simulink model "Boomerang_Simulink_validation_smAoA"  (R2023a)
settings: Solver=ode4  StartTime=0.0  StopTime=t  FixedStep=dt  MaxStep=maxstep  MinStep=minstep
values from neighbouring files (symbols this model uses):
  c = 5e-2    (= 0.05)    [Boomerang_4Wings.m]    (also in Boomerang_4Wings_Titan.m = 0.0488; Boomerang_4Wings_Venus52.m; Boomerang_4Wings_Venus60.m = 0.065; Boomerang_Cropped_Validation.m = 0.0381)
  CDdata = [x_CD, y_CD]    [Boomerang_4Wings.m]    (also in Boomerang_4Wings_Titan.m; Boomerang_4Wings_Venus52.m; Boomerang_4Wings_Venus60.m; Boomerang_Cropped_Validation.m)
  CLdata = [x_CL, y_CL]    [Boomerang_4Wings.m]    (also in Boomerang_4Wings_Titan.m; Boomerang_4Wings_Venus52.m; Boomerang_4Wings_Venus60.m; Boomerang_Cropped_Validation.m)
  CMdata = [x_CM, y_CM]    [Boomerang_4Wings.m]    (also in Boomerang_4Wings_Titan.m; Boomerang_4Wings_Venus52.m; Boomerang_4Wings_Venus60.m; Boomerang_Cropped_Validation.m)
  Eul0 = [0; 0; 0]    [Boomerang_4Wings.m]    (also in Boomerang_4Wings_Titan.m; Boomerang_4Wings_Venus52.m; Boomerang_4Wings_Venus60.m; Boomerang_Cropped_Validation.m)
  g = 9.81    [Boomerang_4Wings.m]    (also in Boomerang_4Wings_Titan.m = 1.35; Boomerang_4Wings_Venus52.m; Boomerang_4Wings_Venus60.m = 8.87; Boomerang_Cropped_Validation.m)
  invJ = inv(J)    [Boomerang_4Wings.m]    (also in Boomerang_4Wings_Titan.m; Boomerang_4Wings_Venus52.m; Boomerang_4Wings_Venus60.m; Boomerang_Cropped_Validation.m)
  invm = inv(m)    [Boomerang_4Wings.m]    (also in Boomerang_4Wings_Titan.m; Boomerang_4Wings_Venus52.m; Boomerang_4Wings_Venus60.m; Boomerang_Cropped_Validation.m)
  invTI0 = transpose(TI0)    [AttitudePlot.m]    (also in AttitudePlot_V0.m = transpose(T); Boomerang_4Wings.m; Boomerang_4Wings_Titan.m; Boomerang_4Wings_Venus52.m)
  invTj = zeros(3,3,nw)    [Boomerang_4Wings.m]    (also in Boomerang_4Wings_Titan.m; Boomerang_4Wings_Venus52.m; Boomerang_4Wings_Venus60.m; Boomerang_Cropped_Validation.m)
  J = J + (Ji(:,:,i))    [Boomerang_4Wings.m]    (also in Boomerang_4Wings_Titan.m = diag(diag(J)); Boomerang_4Wings_Venus52.m; Boomerang_4Wings_Venus60.m; Boomerang_Cropped_Validation.m = [Ixx Ixy Ixz)
  l_integrate = linspace(0,l_blade,n)    [Boomerang_4Wings.m]    (also in Boomerang_4Wings_Titan.m; Boomerang_4Wings_Venus52.m; Boomerang_4Wings_Venus60.m; Boomerang_Cropped_Validation.m = linspace(l_blade_0,l_blade,n))
  m = m_b*eye(3) + m_add    [Boomerang_4Wings.m]    (also in Boomerang_4Wings_Titan.m; Boomerang_4Wings_Venus52.m; Boomerang_4Wings_Venus60.m; Boomerang_Cropped_Validation.m)
  nw = 4    [Boomerang_4Wings.m]    (also in Boomerang_4Wings_Titan.m; Boomerang_4Wings_Venus52.m; Boomerang_4Wings_Venus60.m; Boomerang_Cropped_Validation.m = 3)
  omega0 = [0; 0; 10*pi*2]    [Boomerang_4Wings.m]    (also in Boomerang_4Wings_Titan.m = [0; 0; r*pi*2]; Boomerang_4Wings_Venus52.m; Boomerang_4Wings_Venus60.m; Boomerang_Cropped_Validation.m = [0; 0; r])
  PHI0 = deg2rad(PHI0)    [AttitudePlot.m]    (also in AttitudePlot_V0.m; Boomerang_4Wings.m; Boomerang_4Wings_Titan.m; Boomerang_4Wings_Venus52.m)
  PSI0 = deg2rad(PSI0)    [AttitudePlot.m]    (also in AttitudePlot_V0.m; Boomerang_4Wings.m; Boomerang_4Wings_Titan.m; Boomerang_4Wings_Venus52.m)
  R_pos0 = [0; 0; 1.5]    [Boomerang_4Wings.m]    (also in Boomerang_4Wings_Titan.m; Boomerang_4Wings_Venus52.m; Boomerang_4Wings_Venus60.m; Boomerang_Cropped_Validation.m = [0; 0; 1.8])
  rho = 1.22    [Boomerang_4Wings.m]    (also in Boomerang_4Wings_Titan.m = 5.368; Boomerang_4Wings_Venus52.m = 1.3288004; Boomerang_4Wings_Venus60.m = 0.49007955; Boomerang_Cropped_Validation.m)
  S = pi*R^2    (= 0.196349540849)    [Boomerang_4Wings.m]    (also in Boomerang_4Wings_Titan.m = 0.228; Boomerang_4Wings_Venus52.m; Boomerang_4Wings_Venus60.m = 0.282743338823; Boomerang_Cropped_Validation.m = 0.0651440652648)
  THETA0 = deg2rad(THETA0)    [AttitudePlot.m]    (also in AttitudePlot_V0.m; Boomerang_4Wings.m; Boomerang_4Wings_Titan.m; Boomerang_4Wings_Venus52.m)
  thetaj = 0    [Boomerang_4Wings.m]    (also in Boomerang_4Wings_Titan.m; Boomerang_4Wings_Venus52.m; Boomerang_4Wings_Venus60.m; Boomerang_Cropped_Validation.m = deg2rad(thetaj))
  TI0 = RI01*RI02*RI03    [AttitudePlot.m]    (also in Boomerang_4Wings.m; Boomerang_4Wings_Titan.m; Boomerang_4Wings_Venus52.m; Boomerang_4Wings_Venus60.m)
  Tj = zeros(3,3, nw)    [Boomerang_4Wings.m]    (also in Boomerang_4Wings_Titan.m; Boomerang_4Wings_Venus52.m; Boomerang_4Wings_Venus60.m; Boomerang_Cropped_Validation.m)
  u0 = TI0*U0    [Boomerang_4Wings.m]    (also in Boomerang_4Wings_Titan.m; Boomerang_4Wings_Venus52.m; Boomerang_4Wings_Venus60.m; Boomerang_Cropped_Validation.m)
  v_wind = [0; 0; 0]    [Boomerang_4Wings.m]    (also in Boomerang_4Wings_Titan.m; Boomerang_4Wings_Venus52.m; Boomerang_4Wings_Venus60.m; Boomerang_Cropped_Validation.m)
  x_ac = zeros(3,nw)    [Boomerang_4Wings.m]    (also in Boomerang_4Wings_Titan.m = 0; Boomerang_4Wings_Venus52.m; Boomerang_4Wings_Venus60.m; Boomerang_Cropped_Validation.m)
libraries: simulink_extras x1
settings Model: Creator=dsantis  LastModifiedBy=dsantis

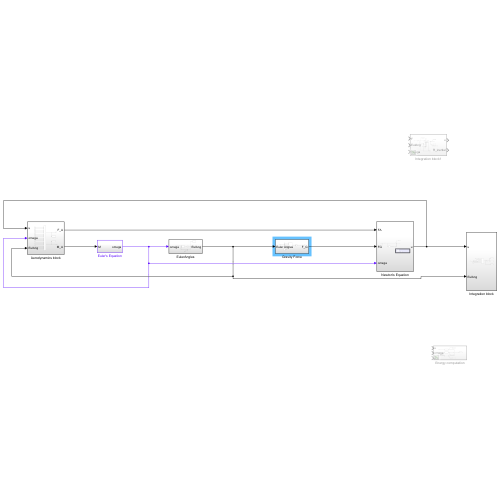
[thumbnail: Simulink's stored preview of the top-level diagram]
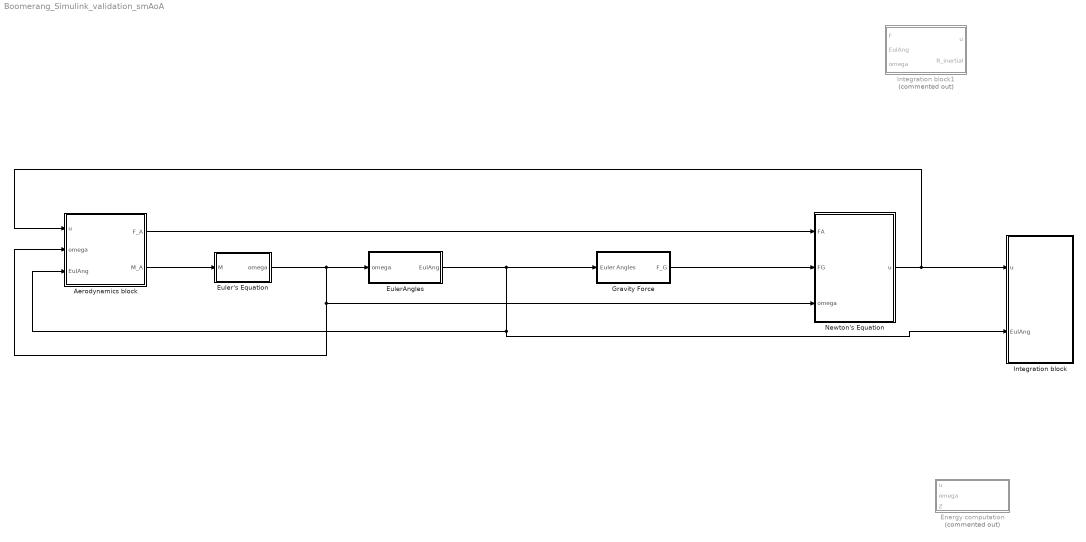
== system Boomerang_Simulink_validation_smAoA ==
  Aerodynamics block : Subsystem
  Energy computation : Subsystem  Commented=on
  Euler's Equation : Subsystem
  EulerAngles : Subsystem
  Gravity Force : Subsystem
  Integration block : Subsystem
  Integration block1 : Subsystem  Commented=on
  Newton's Equation : Subsystem
  wires:
  Euler's Equation/1(omega) -> EulerAngles/1(omega), Aerodynamics block/2(omega), Newton's Equation/3(omega)
  Newton's Equation/1(u) -> Aerodynamics block/1(u), Integration block/1(u)
  Gravity Force/1(F_G) -> Newton's Equation/2(FG)
  Aerodynamics block/2(M_A) -> Euler's Equation/1(M)
  EulerAngles/1(EulAng) -> Aerodynamics block/3(EulAng), Integration block/2(EulAng), Gravity Force/1(Euler Angles)
  Aerodynamics block/1(F_A) -> Newton's Equation/1(FA)

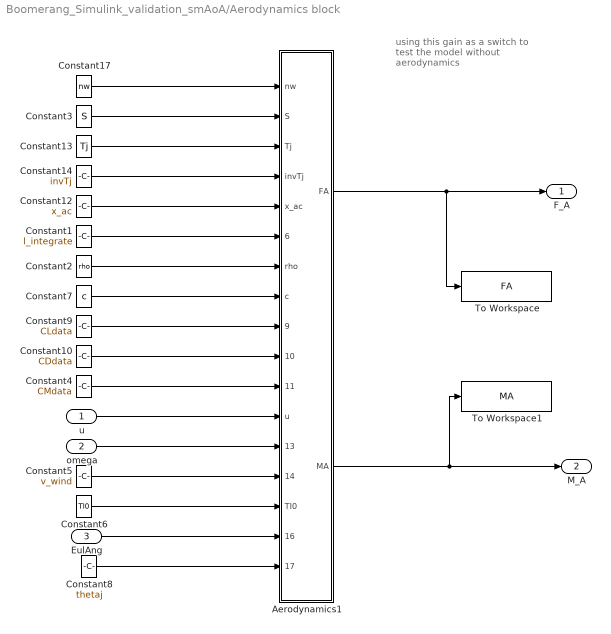
== system Boomerang_Simulink_validation_smAoA/Aerodynamics block ==
  note: using this gain as a switch
      | to test the model without aerodynamics
  u : Inport
  omega : Inport  Port=2
  EulAng : Inport  Port=3
  Aerodynamics1 : MATLAB Function  TreatAsAtomicUnit=on
  Constant1 : Constant  Value=l_integrate
  Constant10 : Constant  Value=CDdata
  Constant12 : Constant  Value=x_ac
  Constant13 : Constant  Value=Tj
  Constant14 : Constant  Value=invTj
  Constant17 : Constant  Value=nw
  Constant2 : Constant  Value=rho
  Constant3 : Constant  Value=S
  Constant4 : Constant  Value=CMdata
  Constant5 : Constant  Value=v_wind
  Constant6 : Constant  Value=TI0
  Constant7 : Constant  Value=c
  Constant8 : Constant  Value=thetaj
  Constant9 : Constant  Value=CLdata
  To Workspace : ToWorkspace  VariableName=FA  SampleTime=-1
  To Workspace1 : ToWorkspace  VariableName=MA  SampleTime=-1
  F_A : Outport
  M_A : Outport  Port=2
  wires:
  u/1 -> Aerodynamics1/12(u)
  Constant2/1 -> Aerodynamics1/7(rho)
  Constant9/1 -> Aerodynamics1/9(CLdata)
  Constant10/1 -> Aerodynamics1/10(CDdata)
  Constant1/1 -> Aerodynamics1/6(l_integrate)
  Constant7/1 -> Aerodynamics1/8(c)
  omega/1 -> Aerodynamics1/13(omega)
  Constant12/1 -> Aerodynamics1/5(x_ac)
  Constant14/1 -> Aerodynamics1/4(invTj)
  Constant13/1 -> Aerodynamics1/3(Tj)
  Constant17/1 -> Aerodynamics1/1(nw)
  Constant3/1 -> Aerodynamics1/2(S)
  Constant4/1 -> Aerodynamics1/11(CMdata)
  Constant5/1 -> Aerodynamics1/14(v_wind)
  Constant6/1 -> Aerodynamics1/15(TI0)
  EulAng/1 -> Aerodynamics1/16(EulAng)
  Constant8/1 -> Aerodynamics1/17(thetaj)
  Aerodynamics1/1(FA) -> To Workspace/1, F_A/1
  Aerodynamics1/2(MA) -> To Workspace1/1, M_A/1

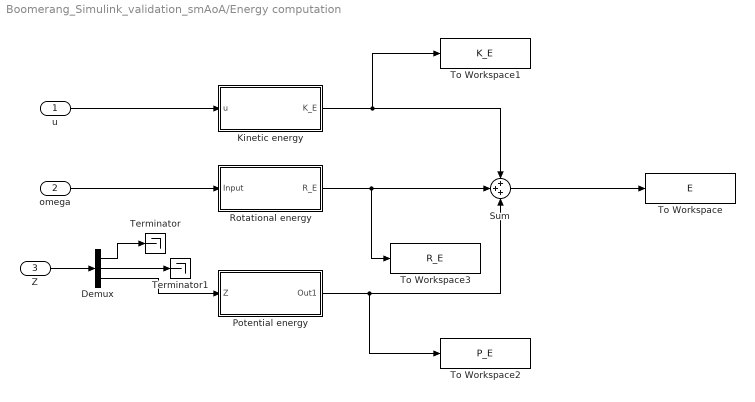
== system Boomerang_Simulink_validation_smAoA/Energy computation ==
  u : Inport
  omega : Inport  Port=2
  Z : Inport  Port=3
  Demux : Demux  Outputs=3
  Kinetic energy : Subsystem
  Potential energy : Subsystem
  Rotational energy : Subsystem
  Sum : Sum  Inputs=+++
  Terminator : Terminator
  Terminator1 : Terminator
  To Workspace : ToWorkspace  VariableName=E  SaveFormat=Timeseries  SampleTime=-1
  To Workspace1 : ToWorkspace  VariableName=K_E  SaveFormat=Timeseries  SampleTime=-1
  To Workspace2 : ToWorkspace  VariableName=P_E  SaveFormat=Timeseries  SampleTime=-1
  To Workspace3 : ToWorkspace  VariableName=R_E  SaveFormat=Timeseries  SampleTime=-1
  wires:
  u/1 -> Kinetic energy/1(u)
  omega/1 -> Rotational energy/1(Input)
  Z/1 -> Demux/1
  Demux/3 -> Potential energy/1(Z)
  Demux/1 -> Terminator/1
  Demux/2 -> Terminator1/1
  Kinetic energy/1(K_E) -> To Workspace1/1, Sum/1
  Rotational energy/1(R_E) -> To Workspace3/1, Sum/2
  Potential energy/1(Out1) -> To Workspace2/1, Sum/3
  Sum/1 -> To Workspace/1

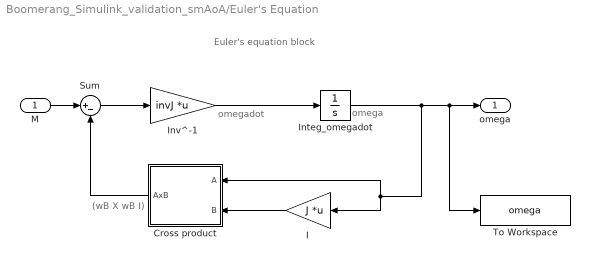
== system Boomerang_Simulink_validation_smAoA/Euler's Equation ==
  note: Euler's equation block
  note: (wB X wB I)
  note: omega
  note: omegadot
  M : Inport
  Cross product : Subsystem
  I : Gain  Gain=J  Multiplication=Matrix(K*u)
  Integ_omegadot : Integrator  InitialCondition=omega0
  Inv^-1 : Gain  Gain=invJ  Multiplication=Matrix(K*u) (u vector)
  Sum : Sum  Inputs=|+-
  To Workspace : ToWorkspace  VariableName=omega  SampleTime=-1
  omega : Outport  VectorParamsAs1DForOutWhenUnconnected=off
  wires:
  Integ_omegadot/1 -> To Workspace/1, omega/1, I/1, Cross product/1(A)
  I/1 -> Cross product/2(B)
  M/1 -> Sum/1
  Sum/1 -> Inv^-1/1
  Inv^-1/1 -> Integ_omegadot/1
  Cross product/1(AxB) -> Sum/2

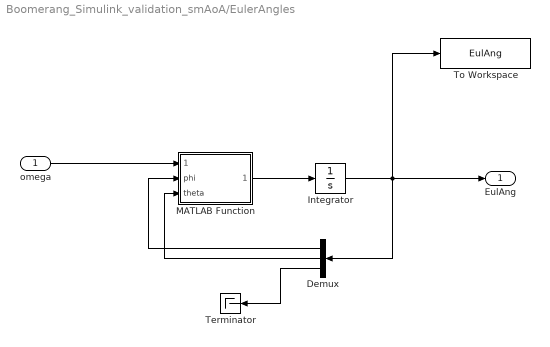
== system Boomerang_Simulink_validation_smAoA/EulerAngles ==
  omega : Inport
  Demux : Demux  Outputs=3
  Integrator : Integrator  InitialCondition=Eul0
  MATLAB Function : MATLAB Function  TreatAsAtomicUnit=on
  Terminator : Terminator
  To Workspace : ToWorkspace  VariableName=EulAng  SampleTime=-1
  EulAng : Outport
  wires:
  omega/1 -> MATLAB Function/1(omega)
  MATLAB Function/1(EulRate) -> Integrator/1
  Integrator/1 -> To Workspace/1, Demux/1, EulAng/1
  Demux/1 -> MATLAB Function/2(phi)
  Demux/2 -> MATLAB Function/3(theta)
  Demux/3 -> Terminator/1

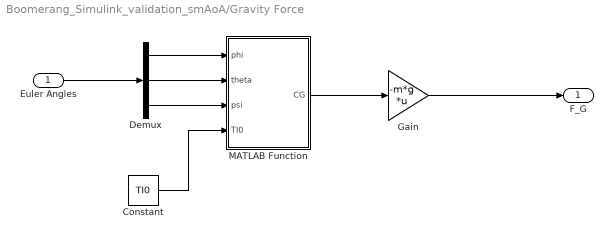
== system Boomerang_Simulink_validation_smAoA/Gravity Force ==
  Euler Angles : Inport
  Constant : Constant  Value=TI0
  Demux : Demux  Outputs=3
  Gain : Gain  Gain=-m*g  Multiplication=Matrix(K*u)
  MATLAB Function : MATLAB Function  TreatAsAtomicUnit=on
  F_G : Outport
  wires:
  Gain/1 -> F_G/1
  Demux/3 -> MATLAB Function/3(psi)
  Demux/2 -> MATLAB Function/2(theta)
  Demux/1 -> MATLAB Function/1(phi)
  MATLAB Function/1(CG) -> Gain/1
  Euler Angles/1 -> Demux/1
  Constant/1 -> MATLAB Function/4(TI0)

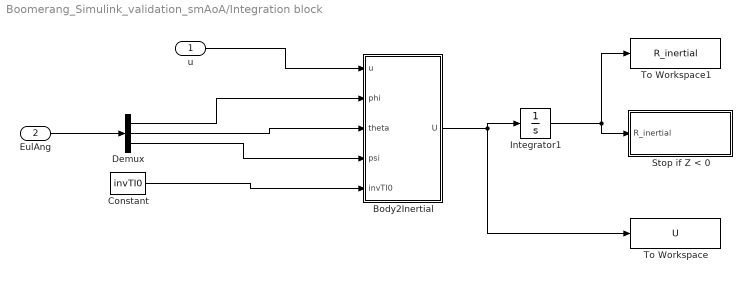
== system Boomerang_Simulink_validation_smAoA/Integration block ==
  u : Inport
  EulAng : Inport  Port=2
  Body2Inertial : MATLAB Function  TreatAsAtomicUnit=on
  Constant : Constant  Value=invTI0
  Demux : Demux  Outputs=3
  Integrator1 : Integrator  InitialCondition=R_pos0
  Stop if Z < 0 : Subsystem
  To Workspace : ToWorkspace  VariableName=U  SampleTime=-1
  To Workspace1 : ToWorkspace  VariableName=R_inertial  SampleTime=-1
  wires:
  Integrator1/1 -> Stop if Z < 0/1(R_inertial), To Workspace1/1
  Body2Inertial/1(U) -> Integrator1/1, To Workspace/1
  Demux/3 -> Body2Inertial/4(psi)
  Demux/2 -> Body2Inertial/3(theta)
  u/1 -> Body2Inertial/1(u)
  Demux/1 -> Body2Inertial/2(phi)
  Constant/1 -> Body2Inertial/5(invTI0)
  EulAng/1 -> Demux/1

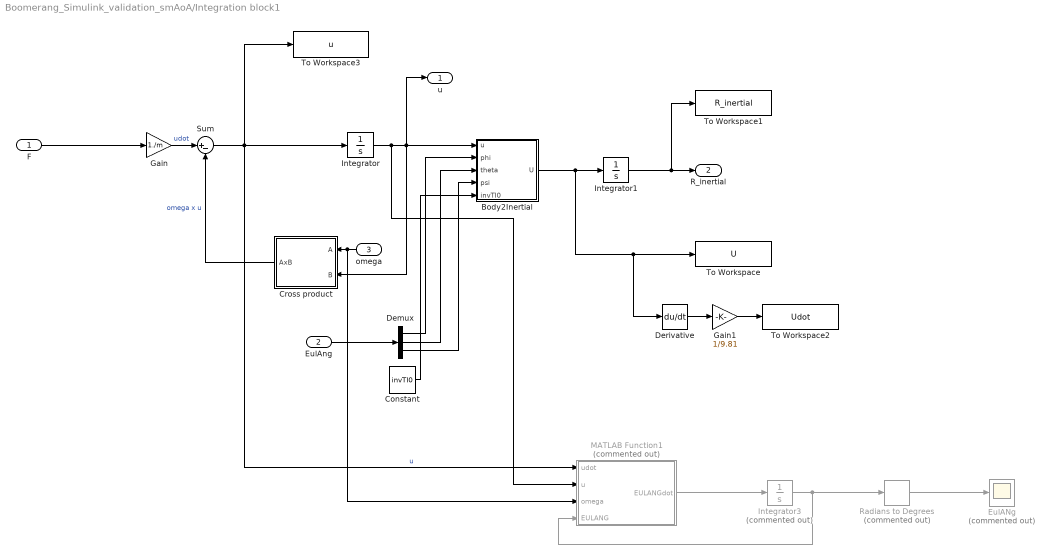
== system Boomerang_Simulink_validation_smAoA/Integration block1 ==
  F : Inport
  EulAng : Inport  Port=2
  omega : Inport  Port=3
  Body2Inertial : MATLAB Function  TreatAsAtomicUnit=on
  Constant : Constant  Value=invTI0
  Cross product : Subsystem
  Demux : Demux  Outputs=3
  Derivative : Derivative
  EulANg : Scope  Commented=on
  Gain : Gain  Gain=1./m
  Gain1 : Gain  Gain=1/9.81
  Integrator : Integrator  InitialCondition=u0
  Integrator1 : Integrator  InitialCondition=R_pos0
  Integrator3 : Integrator  Commented=on  InitialCondition=[PHI0; THETA0; PSI0]
  MATLAB Function1 : MATLAB Function  Commented=on  TreatAsAtomicUnit=on
  Radians to Degrees : simulink_extras/Transformations/Radians to Degrees  Commented=on
  Sum : Sum  Inputs=|+-
  To Workspace : ToWorkspace  VariableName=U  SampleTime=-1
  To Workspace1 : ToWorkspace  VariableName=R_inertial  SampleTime=-1
  To Workspace2 : ToWorkspace  VariableName=Udot  SaveFormat=Timeseries  SampleTime=-1
  To Workspace3 : ToWorkspace  VariableName=u  SampleTime=-1
  u : Outport
  R_inertial : Outport  Port=2
  wires:
  Cross product/1(AxB) -> Sum/2  "omega x u"
  Integrator/1 -> Cross product/2(B), Body2Inertial/1(u), u/1, MATLAB Function1/2(u)
  Integrator1/1 -> To Workspace1/1, R_inertial/1
  Gain/1 -> Sum/1  "udot"
  EulAng/1 -> Demux/1
  Demux/1 -> Body2Inertial/2(phi)
  Demux/2 -> Body2Inertial/3(theta)
  Demux/3 -> Body2Inertial/4(psi)
  Constant/1 -> Body2Inertial/5(invTI0)
  F/1 -> Gain/1
  Body2Inertial/1(U) -> Derivative/1, To Workspace/1, Integrator1/1
  Sum/1 -> To Workspace3/1, MATLAB Function1/1(udot), Integrator/1  "u"
  MATLAB Function1/1(EULANGdot) -> Integrator3/1
  Integrator3/1 -> Radians to Degrees/1, MATLAB Function1/4(EULANG)
  Radians to Degrees/1 -> EulANg/1
  Derivative/1 -> Gain1/1
  Gain1/1 -> To Workspace2/1
  omega/1 -> MATLAB Function1/3(omega), Cross product/1(A)

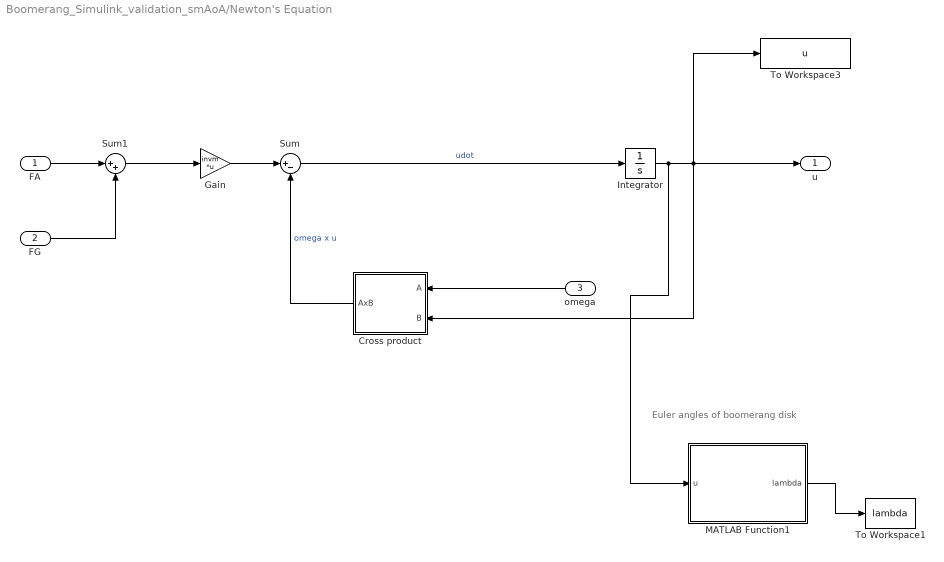
== system Boomerang_Simulink_validation_smAoA/Newton's Equation ==
  note: Euler angles of boomerang disk
  FA : Inport
  FG : Inport  Port=2
  omega : Inport  Port=3
  Cross product : Subsystem
  Gain : Gain  Gain=invm  Multiplication=Matrix(K*u)
  Integrator : Integrator  InitialCondition=u0
  MATLAB Function1 : MATLAB Function  TreatAsAtomicUnit=on
  Sum : Sum  Inputs=|+-
  Sum1 : Sum  Inputs=|++
  To Workspace1 : ToWorkspace  VariableName=lambda  SampleTime=-1
  To Workspace3 : ToWorkspace  VariableName=u  SampleTime=-1
  u : Outport
  wires:
  Cross product/1(AxB) -> Sum/2  "omega x u"
  Gain/1 -> Sum/1
  FA/1 -> Sum1/1
  Sum/1 -> Integrator/1  "udot"
  omega/1 -> Cross product/1(A)
  FG/1 -> Sum1/2
  Sum1/1 -> Gain/1
  Integrator/1 -> MATLAB Function1/1(u), u/1, Cross product/2(B), To Workspace3/1
  MATLAB Function1/1(lambda) -> To Workspace1/1

== system Boomerang_Simulink_validation_smAoA/Energy computation/Kinetic energy ==
  u : Inport
  Gain : Gain  Gain=0.5*m
  Norm : MATLAB Function  TreatAsAtomicUnit=on
  K_E : Outport
  wires:
  u/1 -> Norm/1(u)
  Norm/1(y) -> Gain/1
  Gain/1 -> K_E/1

== system Boomerang_Simulink_validation_smAoA/Energy computation/Potential energy ==
  Z : Inport
  Gain : Gain  Gain=m*g
  Out1 : Outport
  wires:
  Z/1 -> Gain/1
  Gain/1 -> Out1/1

== system Boomerang_Simulink_validation_smAoA/Energy computation/Rotational energy ==
  Input : Inport
  Dot Product : DotProduct  OutDataTypeStr=Inherit: Inherit via internal rule
  Gain : Gain  Gain=0.5*J  Multiplication=Matrix(u*K)
  R_E : Outport
  wires:
  Input/1 -> Dot Product/2, Gain/1
  Gain/1 -> Dot Product/1
  Dot Product/1 -> R_E/1

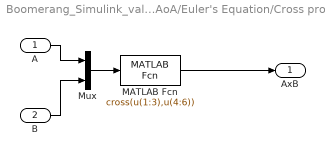
== system Boomerang_Simulink_validation_smAoA/Euler's Equation/Cross product ==
  A : Inport
  B : Inport  Port=2
  MATLAB Fcn : MATLABFcn  MATLABFcn=cross(u(1:3),u(4:6))
  Mux : Mux  Inputs=2
  AxB : Outport  VectorParamsAs1DForOutWhenUnconnected=off
  wires:
  A/1 -> Mux/1
  B/1 -> Mux/2
  Mux/1 -> MATLAB Fcn/1
  MATLAB Fcn/1 -> AxB/1

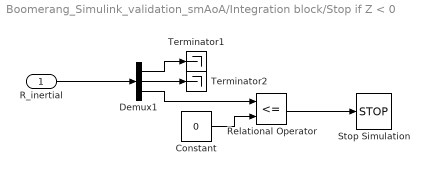
== system Boomerang_Simulink_validation_smAoA/Integration block/Stop if Z < 0 ==
  R_inertial : Inport
  Constant : Constant  Value=0
  Demux1 : Demux  Outputs=3
  Relational Operator : RelationalOperator  Operator=<=  OutDataTypeStr=boolean  RndMeth=Simplest  InputSameDT=off
  Stop Simulation : Stop
  Terminator1 : Terminator
  Terminator2 : Terminator
  wires:
  R_inertial/1 -> Demux1/1
  Demux1/1 -> Terminator1/1
  Demux1/3 -> Relational Operator/1
  Demux1/2 -> Terminator2/1
  Constant/1 -> Relational Operator/2
  Relational Operator/1 -> Stop Simulation/1

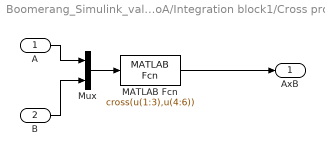
== system Boomerang_Simulink_validation_smAoA/Integration block1/Cross product ==
  A : Inport
  B : Inport  Port=2
  MATLAB Fcn : MATLABFcn  MATLABFcn=cross(u(1:3),u(4:6))
  Mux : Mux  Inputs=2
  AxB : Outport  VectorParamsAs1DForOutWhenUnconnected=off
  wires:
  A/1 -> Mux/1
  B/1 -> Mux/2
  Mux/1 -> MATLAB Fcn/1
  MATLAB Fcn/1 -> AxB/1

== system Boomerang_Simulink_validation_smAoA/Newton's Equation/Cross product ==
  A : Inport
  B : Inport  Port=2
  MATLAB Fcn : MATLABFcn  MATLABFcn=cross(u(1:3),u(4:6))
  Mux : Mux  Inputs=2
  AxB : Outport  VectorParamsAs1DForOutWhenUnconnected=off
  wires:
  A/1 -> Mux/1
  B/1 -> Mux/2
  Mux/1 -> MATLAB Fcn/1
  MATLAB Fcn/1 -> AxB/1

== matlab function Boomerang_Simulink_validation_smAoA/Aerodynamics block/Aerodynamics1 ==
  settings: updateMethod=DISCRETE
  data: nw input; S input; Tj input; invTj input; x_ac input; l_integrate input; rho input; c input; CLdata input; CDdata input; CMdata input; u input; omega input; v_wind input; TI0 input; EulAng input; FA output; thetaj input; MA output
function [FA, MA] = fcn(nw, S, Tj, invTj, x_ac, l_integrate, rho, c, CLdata, CDdata, CMdata,u, omega, v_wind, TI0, EulAng, thetaj)

phi = EulAng(1);
theta = EulAng(2);
psi = EulAng(3);

R01 = [1, 0, 0; 0, cos(phi), sin(phi); 0, -sin(phi), cos(phi)];
R02 = [cos(theta), 0, -sin(theta); 0, 1, 0; sin(theta), 0, cos(theta)];
R03 = [cos(psi), sin(psi), 0; -sin(psi), cos(psi), 0; 0, 0, 1];
T0 = R01*R02*R03;

persistent flag v_bar
if isempty(flag)
    flag = false;
    v_bar = 0;
end

v_ind = [0; 0; -v_bar];

FA = [0; 0; 0];
MA = [0;0;0];

l_b = l_integrate(end);
Cl0 =  0.3484;
Cd0 = 0.02;
d1 = 1.5;
Cla = 5.7;
Cm0 = -0.09;
Cma = -0.27;
v_ind = [zeros(size(l_integrate)), zeros(size(l_integrate)), v_bar*(1+1.2*l_integrate./(l_integrate(end)))]';
% Piecewise linear fit for CL
C_L = @(alpha) interp1(CLdata(:,1), CLdata(:,2), alpha, 'linear', 'extrap');

% Piecewise linear fit for CD
C_D = @(alpha) interp1(CDdata(:,1), CDdata(:,2), alpha, 'linear', 'extrap');

 % Piecewise linear fit for CM
C_M = @(alpha) interp1(CMdata(:,1), CMdata(:,2), alpha, 'linear', 'extrap');
n = length(l_integrate);

for i = 1:nw
    
    rA = [x_ac.*ones(1,n); zeros(1,n); zeros(1,n)] + invTj(:,:,i)*[zeros(1,n); l_integrate'; zeros(1,n)];
    w = Tj(:,:,i)*( (-u -cross(omega.*ones(3,n), rA)) + v_ind + T0*TI0*v_wind);
    alpha = (atan2(w(3,:),w(1,:))) + thetaj;

    w2 = w(1,:).^2 + w(3,:).^2;

    l = (0.5*rho*c).*w2.*C_L(alpha);
    d = (0.5*rho*c).*w2.*C_D(alpha);
    m_eta = (0.5*rho*c^2).*w2.*C_M(alpha);

    int_funx = -l.*sin(alpha) + d.*cos(alpha);
    int_funz = l.*cos(alpha) + d.*sin(alpha);

    funM = cross([zeros(1,n); l_integrate'; zeros(1,n)], [-int_funx; zeros(1,n); int_funz]);
    int_funMx = funM(1,:);
    int_funMy = m_eta; 
    int_funMz = funM(3,:);
    % 
    FxjA = trapz(l_integrate,int_funx);
    FzjA = trapz(l_integrate,int_funz);
    % 
    MxjA = trapz(l_integrate,int_funMx);
    MyjA = trapz(l_integrate,int_funMy);
    MzjA = trapz(l_integrate,int_funMz);
    v = Tj(:,:,i)*(-u + v_ind);
    FxjA = 1/2*rho*c*( (-v(3)*Cl0*(v(1)*l_b+omega(3)*l_b^2/2)+Cd0*(v(1)^2*l_b+v(1)*omega(3)*l_b^2+omega(3)^2*l_b^3/3)) );
    FzjA = 1/2*rho*c*( (v(1)^2*l_b + v(1)*omega(3)*l_b^2 + omega(3)^2*l_b^3/3)*Cl0 + Cla*v(3)*(v(1)*l_b+omega(3)*l_b^2/2) + 0*v(3)*Cd0*(v(1)^2*l_b + v(1)*omega(3)*l_b^2 + omega(3)^2*l_b^3/3));

    % MxjA = 1.2*1/2*rho*c*( Cl0*(v(1)^2*l_b^2/2 + 2/3*v(1)*omega(3)*l_b^3 + omega(3)^2*l_b^4/4) + Cla*v(3)*(v(1)*l_b^2/2 + omega(3)*l_b^3/3) + v(3)*Cd0*(v(1)^2*l_b^2/2 + 2/3*v(1)*omega(3)*l_b^3 + omega(3)^2*l_b^4/4) + d1*v(3)^2*l_b);
    % MyjA = 1/2*rho*c^2*((v(1)^2*l_b + omega(3)*v(1)*l_b^2 + omega(3)^2*l_b^3/3)*Cm0 + (v(1)*l_b + omega(3)*l_b^2/2)*Cma*v(3));
    % MzjA = -1/2*rho*c*( v(3)*Cl0*(v(1)*l_b^2/2 + omega(3)*l_b^3/3) - Cd0*(v(1)^2*l_b^2/2 + 2/3*v(1)*omega(3)*l_b^3/3 + omega(3)^2*l_b^4/4) );

    FjA = [FxjA; 0; FzjA];
    FA = FA + invTj(:,:,i)*FjA;

    MjA = [MxjA'; MyjA; MzjA];
    MA = MA + invTj(:,:,i)*MjA + cross([x_ac; 0; 0], invTj(:,:,1)*FjA);
end
f = @(v_ind) v_ind - FA(3)/(2*rho*S*sqrt(norm([u(1) u(2)])^2 + (u(3)-v_ind)^2));
v_bar = fzero(f,0);

== matlab function Boomerang_Simulink_validation_smAoA/Gravity Force/MATLAB Function ==
  data: phi input; theta input; psi input; CG output; TI0 input
function CG = fcn(phi, theta, psi, TI0)
R01 = [
    1, 0, 0;
    0, cos(phi), sin(phi);
    0, -sin(phi), cos(phi)
    ];
R02 = [
    cos(theta), 0, -sin(theta);
    0, 1, 0;
    sin(theta), 0, cos(theta)
];
R03 = [
    cos(psi), sin(psi), 0;
    -sin(psi), cos(psi), 0;
    0, 0, 1
];
T0 = R01*R02*R03;

CG = T0*TI0*[0; 0; 1];

== matlab function Boomerang_Simulink_validation_smAoA/Integration block/Body2Inertial ==
  data: u input; U output; phi input; theta input; psi input; invTI0 input
function U   = fcn(u, phi, theta, psi, invTI0)
R01 = [
    1, 0, 0;
    0, cos(phi), sin(phi);
    0, -sin(phi), cos(phi)
    ];
R02 = [
    cos(theta), 0, -sin(theta);
    0, 1, 0;
    sin(theta), 0, cos(theta)
];
R03 = [
    cos(psi), sin(psi), 0;
    -sin(psi), cos(psi), 0;
    0, 0, 1
];
T0 = R01*R02*R03;
invT0 = transpose(T0);

U = invTI0*invT0*u;

== matlab function Boomerang_Simulink_validation_smAoA/EulerAngles/MATLAB Function ==
  data: omega input; EulRate output; phi input; theta input
function EulRate = fcn(omega, phi, theta)

phidot = omega(1) + omega(2)*sin(phi)*tan(theta) + omega(3)*cos(phi)*tan(theta);
thetadot = omega(2)*cos(phi) - omega(3)*sin(phi);
psidot = omega(2)*sin(phi)/cos(theta) + omega(3)*cos(phi)/cos(theta);

EulRate = [phidot; thetadot; psidot];

== matlab function Boomerang_Simulink_validation_smAoA/Energy computation/Kinetic energy/Norm ==
  data: u input; y output
function y = fcn(u)

y = norm(u)^2;

== matlab function Boomerang_Simulink_validation_smAoA/Integration block1/Body2Inertial ==
  data: u input; U output; phi input; theta input; psi input; invTI0 input
function U = fcn(u, phi, theta, psi, invTI0)
R01 = [
    1, 0, 0;
    0, cos(phi), sin(phi);
    0, -sin(phi), cos(phi)
    ];
R02 = [
    cos(theta), 0, -sin(theta);
    0, 1, 0;
    sin(theta), 0, cos(theta)
];
R03 = [
    cos(psi), sin(psi), 0;
    -sin(psi), cos(psi), 0;
    0, 0, 1
];
T0 = R01*R02*R03;
invT0 = transpose(T0);
U = invTI0*invT0*u;

== matlab function Boomerang_Simulink_validation_smAoA/Newton's Equation/MATLAB Function1 ==
  data: u input; lambda output
function lambda  = fcn(u)
% udotx = udot(1);
% udoty = udot(2);

ux = u(1);
uy = u(2);

% p = omega(1);
% q = omega(2);
% r = omega(3);
% 
% PHI = EULANG(1);
% THETA = EULANG(2);
% 
% rn = r + (udoty*ux - udotx*uy)/(ux^2 + uy^2);

lambda = -atan2(uy,ux);

% PHIdot = (p*cos(lambda) - q*sin(lambda)) + (p*sin(lambda) + q*cos(lambda))*sin(PHI)*tan(THETA) + ...
%     rn*cos(PHI)*tan(THETA);
% THETAdot = (p*sin(lambda) + q*cos(lambda))*cos(PHI) - rn*sin(PHI);
% PSIdot = (p*sin(lambda) + q*cos(lambda))*sin(PHI)/cos(THETA) + rn*cos(PHI)/cos(THETA);

% EULANGdot = [PHIdot; THETAdot; PSIdot];

== matlab function Boomerang_Simulink_validation_smAoA/Integration block1/MATLAB Function1 ==
  data: udot input; u input; EULANGdot output; omega input; EULANG input
function EULANGdot = fcn(udot, u, omega, EULANG)
udotx = udot(1);
udoty = udot(2);

ux = u(1);
uy = u(2);

p = omega(1);
q = omega(2);
r = omega(3);

PHI = EULANG(1);
THETA = EULANG(2);

rn = r + (udoty*ux - udotx*uy)/(ux^2 + uy^2);
lambda = -tan(uy/ux);

PHIdot = (p*cos(lambda) - q*sin(lambda)) + (p*sin(lambda) + q*cos(lambda))*sin(PHI)*tan(THETA) + ...
    rn*cos(PHI)*tan(THETA);
THETAdot = (p*sin(lambda) + q*cos(lambda))*cos(PHI) - rn*sin(PHI);
PSIdot = (p*sin(lambda) + q*cos(lambda))*sin(PHI)/cos(THETA) + rn*cos(PHI)/cos(THETA);

EULANGdot = [PHIdot; THETAdot; PSIdot];
